simulink model "Model_02"  (R2014a)
settings: Solver=ode3  SolverMode=SingleTasking  StartTime=0.0  StopTime=totalSimulationTime  FixedStep=t_Sim  RelTol=1e-3
model workspace: external: MATLAB File Init_Model_02_Simulink.m (data not in the file)
values from neighbouring files (symbols this model uses):
  Cov_nu = [0.005 0 0 0 ... (first row only)    [InitOOSM.m]    (also in InitSIL.m; Init_Model_02_Simulink.m = 5e-3*eye(4,4); Init_Model_02_Simulink_SIL1.m)
  Cov_r = [0.003 0 0 ... (first row only)    [InitOOSM.m]    (also in InitSIL.m; Init_Model_02_Simulink.m = 3e-3*eye(3,3); Init_Model_02_Simulink_SIL1.m)
  e_force_x = 0    [InitOOSM.m]    (also in InitSIL.m; Init_Model_02_Simulink.m; Init_Model_02_Simulink_SIL1.m)
  e_force_y = 0    [InitOOSM.m]    (also in InitSIL.m; Init_Model_02_Simulink.m; Init_Model_02_Simulink_SIL1.m)
  e_force_z = 0    [InitOOSM.m]    (also in InitSIL.m; Init_Model_02_Simulink.m; Init_Model_02_Simulink_SIL1.m)
  ita = [0.5;0.5;0.5;0.5]    [InitOOSM.m]    (also in InitSIL.m; Init_Model_02_Simulink.m = [0.12;0.05;-0.15;0.98]; Init_Model_02_Simulink_SIL1.m)
  n = 0.00    (= 0)    [InitOOSM.m]    (also in InitSIL.m; Init_Model_02_Simulink_SIL1.m)
  p_x = 0.75    [InitOOSM.m]    (also in InitSIL.m; Init_Model_02_Simulink.m; Init_Model_02_Simulink_SIL1.m)
  p_y = 0.125    [InitOOSM.m]    (also in InitSIL.m; Init_Model_02_Simulink.m; Init_Model_02_Simulink_SIL1.m)
  p_z = -0.8    [InitOOSM.m]    (also in InitSIL.m; Init_Model_02_Simulink.m; Init_Model_02_Simulink_SIL1.m)
  parameter_gravitation = 3.986005E+14    (= 398600500000000)    [InitOOSM.m]    (also in InitSIL.m; Init_Model_02_Simulink_SIL1.m)
  rho = [0.04;0;0.3]    [InitOOSM.m]    (also in InitSIL.m; Init_Model_02_Simulink.m = [0.2;0.1;0.05]; Init_Model_02_Simulink_SIL1.m)
  rho_c = [-0.00017;   -0.9780;   -0.1854]    [InitOOSM.m]    (also in InitSIL.m = [0.00036;   -0.9865;   -0.1854]; Init_Model_02_Simulink.m = [0;0;0.9]; Init_Model_02_Simulink_SIL1.m = [0.00036;   -0.9865;   -0.1854])
  sig_f = 2E-6    (= 2e-06)    [InitOOSM.m]    (also in InitSIL.m; Init_Model_02_Simulink.m; Init_Model_02_Simulink_SIL1.m)
  sig_tau = 2.5E-5    (= 2.5e-05)    [InitOOSM.m]    (also in InitSIL.m; Init_Model_02_Simulink.m; Init_Model_02_Simulink_SIL1.m)
  t_delta = 0.2    [InitOOSM.m]    (also in InitSIL.m; Init_Model_02_Simulink_SIL1.m)
  t_Kalman = 0.01    [InitOOSM.m]    (also in InitSIL.m; Init_Model_02_Simulink_SIL1.m)
  t_Sim = 0.001    [InitOOSM.m]    (also in InitSIL.m; Init_Model_02_Simulink_SIL1.m)
  tau_1 = 0    [InitOOSM.m]    (also in InitSIL.m; Init_Model_02_Simulink.m; Init_Model_02_Simulink_SIL1.m)
  tau_2 = 0    [InitOOSM.m]    (also in InitSIL.m; Init_Model_02_Simulink.m; Init_Model_02_Simulink_SIL1.m)
  tau_3 = 0    [InitOOSM.m]    (also in InitSIL.m; Init_Model_02_Simulink.m; Init_Model_02_Simulink_SIL1.m)
  X_a_0 = [0; 0; 0; 1; 0; 0; 0; 0; 0; 0; 0; 0; 0;0;0;0;0;0;0;1]    [InitOOSM.m]    (also in InitSIL.m = [0; 0; 0; 1; 0; 0; 0; 0; 0; 0; 0; 0; 0]; Init_Model_02_Simulink.m = [q_1_0;q_2_0;q_3_0;q_0_0;om_x_0;om_y_0;om_z_0;r_x_0;r_y_0;r_; Init_Model_02_Simulink_SIL1.m = [0;0;0.707;0.707;0.2;-0.02;0.0001;0.02;-1.80;0.50;-0.05;0.00)
undefined symbols (not defined in the file or in its folder): DiscIntNeverNeededParam, gray
libraries: simulink x7, aerolibtransform2 x2, visionsinks x1
(part 1 of 3)
settings Model: PauseTimes=3  NumberOfSteps=100  Creator=Iseberg-2  LastModifiedBy=Iseberg
settings SolverCC: AutoInsertRateTranBlk=on
settings DebuggingCC: UnderspecifiedInitializationDetection=Classic  CheckExecutionContextPreStartOutputMsg=on  CheckExecutionContextRuntimeOutputMsg=on

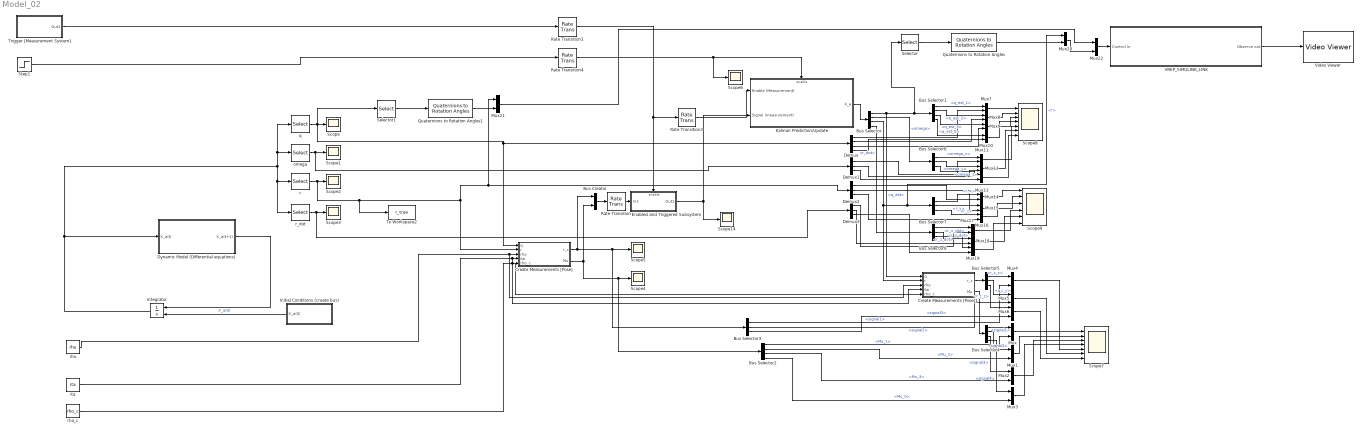
== system Model_02 ==
  Bus Creator : BusCreator  Inputs=2
  Bus Selector : BusSelector  OutputSignals=q_est,omega,r,r_dot
  Bus Selector1 : BusSelector  OutputSignals=q_est_1,q_est_2,q_est_3,q_est_0
  Bus Selector2 : BusSelector  OutputSignals=Mu_1,Mu_2,Mu_3,Mu_0
  Bus Selector3 : BusSelector
  Bus Selector4 : BusSelector  OutputSignals=signal1,signal2,signal3,signal4
  Bus Selector5 : BusSelector  OutputSignals=r_c_x,r_c_y,r_c_z
  Bus Selector6 : BusSelector  OutputSignals=omega_x,omega_y,omega_z
  Bus Selector7 : BusSelector  OutputSignals=r_x,r_y,r_z
  Bus Selector8 : BusSelector  OutputSignals=r_x_dot,r_y_dot,r_z_dot
  Create Measurements [Pose] : Subsystem
  Create Measurements [Pose]1 : Subsystem
  Demux : Demux
  Demux1 : Demux  Outputs=3
  Demux2 : Demux  Outputs=3
  Demux3 : Demux  Outputs=3
  Dynamic Model (Differential equations) : Subsystem
  Enabled and Triggered Subsystem : Subsystem  TreatAsAtomicUnit=on
  Initial Conditions (create bus) : Subsystem
  Integrator : Integrator  InitialConditionSource=external
  Kalman Prediction/Update : Subsystem  TreatAsAtomicUnit=on
  Mux{,1..22} (23 alike) : Mux  Inputs=2
  Quaternions to Rotation Angles : aerolibtransform2/Quaternions to Rotation Angles  rotationOrder=ZYX
  Quaternions to Rotation Angles1 : aerolibtransform2/Quaternions to Rotation Angles  rotationOrder=ZYX
  Rate Transition : RateTransition  OutPortSampleTime=t_delta
  Rate Transition1 : RateTransition  OutPortSampleTime=t_Kalman
  Rate Transition3 : RateTransition  OutPortSampleTime=t_delta
  Rate Transition4 : RateTransition  OutPortSampleTime=t_Kalman
  Scope{,1..6,14} (8 alike) : Scope
      Scope settings: ShowLegends=on  YMin=-1  YMax=1  MaxDataPoints=100000
      Scope1 settings: ShowLegends=on  TimeRange=40
      Scope14 settings: SaveName=ScopeData31
      Scope2 settings: ShowLegends=on  SaveName=ScopeData2
      Scope3 settings: ShowLegends=on  SaveName=ScopeData3
      Scope4 settings: ShowLegends=on  TimeRange=40  SaveName=ScopeData4
      Scope5 settings: ShowLegends=on  SaveName=ScopeData5
      Scope6 settings: YMin=0.95  YMax=1.05  SaveName=ScopeData7
  Scope7 : Scope  NumInputPorts=7
      settings: ShowLegends=on  TimeRange=200  YMin=-1~-5~-5~-5~-5~-5~-5  YMax=1~5~5~5~5~5~5  SaveName=ScopeData9
  Scope8 : Scope  NumInputPorts=7
      settings: ShowLegends=on  TimeRange=200  YMin=-1~-1~-1~-1~0.4~-0.4~-1  YMax=0.75~1~1~0.75~0.95~0.4~1  SaveName=ScopeData24
  Scope9 : Scope  NumInputPorts=6
      settings: ShowLegends=on  TimeRange=200  YMin=-1~-5~-5~-5~-5~-5  YMax=1~5~5~5~5~5  SaveName=ScopeData11
  Selector : Selector  InputPortWidth=4  Indices=[4 1 2 3]
  Selector1 : Selector  InputPortWidth=4  Indices=[4 1 2 3]
  Step1 : Step  Time=0  SampleTime=t_Sim
  To Workspace2 : ToWorkspace  VariableName=r_true  SaveFormat=Timeseries  SampleTime=-1
  Trigger [Measurement System] : Subsystem
  VREP_SIMULINK_LINK : Subsystem  mask{ObjectsInScene=DefaultCamera, m_ControlObjects={ 'Satellite_Model','Parent';'Satellite_Model_Est','Parent'}, m_InitialControllablePose={[X_a_0_sim.X_a_0_Model_02(9:11);X_a_0_sim.eulerAngles_X_a_0'];zeros(6,1)}, m_ObserveObjects={ 'Vision_sensor','Image' }, sceneFileName=C:\Program Files (x86)\V-REP3\V-REP_PRO_EDU\scenes\Scene_MotionEstimation_1.ttt, OutPortSampleTime=0.05}
      mask prompts: ObjectsInScene "Objects present in scene:"; m_ControlObjects "Control Objects:"; m_InitialControllablePose "Initial Pose:"; m_ObserveObjects "Observing Objects:"; sceneFileName "Scene filename:"; OutPortSampleTime "VREP Sample time [s]"
      mask TypeOptions ObjectsInScene: DefaultCamera | DefaultXViewCamera | DefaultYViewCamera | DefaultZViewCamera | XYZCameraProxy | DefaultNXViewCamera | DefaultNYViewCamera | DefaultNZViewCamera | DefaultLightA | DefaultLightB | DefaultLightC | DefaultLightD | ResizableFloor_5_25 | ResizableFloor_5_25_element | ResizableFloor_5_25_visibleElement | Satellite_Model | Satellite_Model_Est | redundantRobot0 | redundantRob_manipSphere0 | redundantRob_target0 | redundantRob_link8 | redundantRob_joint8 | Rectangle0 | redundantRob_joint9 | Cylinder4 | redundantRob_joint10 | Rectangle5 | redundantRob_joint11 | Cylinder5 | redundantRob_joint12 | Rectangle6 | redundantRob_joint13 | Cylinder6 | redundantRob_joint14 | Rectangle7 | redundantRob_link9 | redundantRob_tip0 | redundantRob_link10 | redundantRob_link11 | redundantRob_link12 | redundantRob_link13 | redundantRob_link14 | redundantRob_link15 | Vision_sensor
      mask TypeOptions m_ControlObjects: VREP_SIMULINK_SYS_OBJ/m_ControlObjects
      mask TypeOptions m_InitialControllablePose: VREP_SIMULINK_SYS_OBJ/m_InitialControllablePose
      mask TypeOptions m_ObserveObjects: VREP_SIMULINK_SYS_OBJ/m_ObserveObjects
      mask TypeOptions sceneFileName: VREP_SIMULINK_SYS_OBJ/sceneFileName
      mask TypeOptions OutPortSampleTime: Rate Transition/OutPortSampleTime | Rate Transition1/OutPortSampleTime
      mask DialogControl Control1 Prompt: V-REP Simulink LINK block settings
      mask DialogControl Container8 Prompt: V-REP settings
      mask Display:
      | image('C:\Users\Iseberg\Pictures\Vrep_image.png')
      | port_label('input',1,'Control in');
      | port_label('output',1,'Observe out');
  Video Viewer : visionsinks/Video Viewer  inputType=Obsolete7b  imagePorts=One multidimensional signal  useColorMap=off  colormapValue=gray(256)  specRange=off  minInputVal=0  maxInputVal=255  FigPos=[9 718 1350 611]  AxisZoom=on  trueSizedOnce=off  OpenAtMdlStart=on  DefaultConfigurationName=vipscopes.VideoViewerScopeCfg
  ita : Constant  Value=ita
  omega : Selector  NumberOfDimensions=2  InputPortWidth=3  IndexOptions=Index vector (dialog),Index vector (dialog)  Indices=[5 6 7],1  OutputSizes=1,1
  q : Selector  NumberOfDimensions=2  InputPortWidth=3  IndexOptions=Index vector (dialog),Index vector (dialog)  Indices=[1 2 3 4],1  OutputSizes=1,1
  r : Selector  NumberOfDimensions=2  InputPortWidth=3  IndexOptions=Index vector (dialog),Index vector (dialog)  Indices=[8 9 10],1  OutputSizes=1,1
  r_dot : Selector  NumberOfDimensions=2  InputPortWidth=3  IndexOptions=Index vector (dialog),Index vector (dialog)  Indices=[11 12 13],1  OutputSizes=1,1
  "rho " : Constant  Value=rho
  rho_c : Constant  Value=rho_c
  wires:
  Initial Conditions (create bus)/1("X_a(0) ") -> Integrator/2  "X_a(0)"
  Dynamic Model (Differential equations)/1(X_a(t+1)) -> Integrator/1
  omega/1 -> Demux1/1, Scope1/1
  r_dot/1 -> Demux3/1, Scope3/1
  Integrator/1 -> r_dot/1, r/1, q/1, omega/1, Dynamic Model (Differential equations)/1(X_a(t))
  "rho "/1 -> Create Measurements [Pose]1/3(rho), Create Measurements [Pose]/3(rho)
  ita/1 -> Create Measurements [Pose]1/4(ita), Create Measurements [Pose]/4(ita)
  rho_c/1 -> Create Measurements [Pose]1/5("rho_c "), Create Measurements [Pose]/5("rho_c ")
  Create Measurements [Pose]/1(r_c) -> Bus Selector3/1, Scope5/1, Bus Creator/1
  Create Measurements [Pose]/2(Mu) -> Bus Creator/2, Bus Selector2/1, Scope4/1
  Bus Creator/1 -> Rate Transition/1
  Trigger [Measurement System]/1(Out1) -> Rate Transition1/1
  Kalman Prediction/Update/1(X_a) -> Bus Selector/1
  Bus Selector/1 -> Selector/1, Bus Selector1/1, Create Measurements [Pose]1/1(q)  "<q_est>"
  Bus Selector/3 -> Create Measurements [Pose]1/2(r), Mux20/1, Bus Selector7/1  "<r>"
  Step1/1 -> Rate Transition4/1
  Create Measurements [Pose]1/2(Mu) -> Bus Selector4/1
  Rate Transition1/1 -> Rate Transition3/1, Enabled and Triggered Subsystem/Enable
  Rate Transition3/1 -> Kalman Prediction/Update/1(Enable (Measurement))
  Rate Transition4/1 -> Scope6/1, Kalman Prediction/Update/Enable
  Rate Transition/1 -> Enabled and Triggered Subsystem/1(In1)
  Enabled and Triggered Subsystem/1(Out1) -> Kalman Prediction/Update/2(Signal (measurement)), Scope14/1
  Bus Selector2/1 -> Mux/2  "<Mu_1>"
  Bus Selector4/1 -> Mux/1  "<signal1>"
  Bus Selector4/2 -> Mux1/1  "<signal2>"
  Bus Selector2/2 -> Mux1/2  "<Mu_2>"
  Bus Selector4/3 -> Mux2/1  "<signal3>"
  Bus Selector2/3 -> Mux2/2  "<Mu_3>"
  Bus Selector4/4 -> Mux3/1  "<signal4>"
  Bus Selector2/4 -> Mux3/2  "<Mu_0>"
  Mux/1 -> Scope7/1
  Mux1/1 -> Scope7/2
  Mux2/1 -> Scope7/3
  Mux3/1 -> Scope7/4
  Create Measurements [Pose]1/1(r_c) -> Bus Selector5/1
  Bus Selector5/1 -> Mux4/1  "<r_c_x>"
  Bus Selector3/1 -> Mux4/2  "<signal1>"
  Bus Selector5/2 -> Mux5/1  "<r_c_y>"
  Bus Selector3/2 -> Mux5/2  "<signal2>"
  Bus Selector5/3 -> Mux6/1  "<r_c_z>"
  Bus Selector3/3 -> Mux6/2  "<signal3>"
  Mux4/1 -> Scope7/5
  Mux5/1 -> Scope7/6
  Mux6/1 -> Scope7/7
  Bus Selector1/1 -> Mux7/1  "<q_est_1>"
  Mux7/1 -> Scope8/1
  Demux/1 -> Mux7/2
  q/1 -> Selector1/1, Create Measurements [Pose]/1(q), Demux/1, Scope/1
  Bus Selector1/2 -> Mux8/1  "<q_est_2>"
  Demux/2 -> Mux8/2
  Bus Selector1/3 -> Mux9/1  "<q_est_3>"
  Demux/3 -> Mux9/2
  Bus Selector1/4 -> Mux10/1  "<q_est_0>"
  Demux/4 -> Mux10/2
  Mux8/1 -> Scope8/2
  Mux9/1 -> Scope8/3
  Mux10/1 -> Scope8/4
  Bus Selector/2 -> Bus Selector6/1  "<omega>"
  Bus Selector6/1 -> Mux11/1  "<omega_x>"
  Demux1/1 -> Mux11/2
  Bus Selector6/2 -> Mux12/1  "<omega_y>"
  Demux1/2 -> Mux12/2
  Bus Selector6/3 -> Mux13/1  "<omega_z>"
  Demux1/3 -> Mux13/2
  Mux11/1 -> Scope8/5
  Mux12/1 -> Scope8/6
  Mux13/1 -> Scope8/7
  Bus Selector7/1 -> Mux14/1  "<r_x>"
  Demux2/1 -> Mux14/2
  Bus Selector7/2 -> Mux15/1  "<r_y>"
  Demux2/2 -> Mux15/2
  Bus Selector7/3 -> Mux16/1  "<r_z>"
  Demux2/3 -> Mux16/2
  Mux14/1 -> Scope9/1
  Mux15/1 -> Scope9/2
  Mux16/1 -> Scope9/3
  Bus Selector/4 -> Bus Selector8/1  "<r_dot>"
  Bus Selector8/1 -> Mux17/1  "<r_x_dot>"
  Demux3/1 -> Mux17/2
  Bus Selector8/2 -> Mux18/1  "<r_y_dot>"
  Demux3/2 -> Mux18/2
  Bus Selector8/3 -> Mux19/1  "<r_z_dot>"
  Demux3/3 -> Mux19/2
  Mux17/1 -> Scope9/4
  Mux18/1 -> Scope9/5
  Mux19/1 -> Scope9/6
  Selector/1 -> Quaternions to Rotation Angles/1
  Selector1/1 -> Quaternions to Rotation Angles1/1
  Quaternions to Rotation Angles1/1 -> Mux21/2
  VREP_SIMULINK_LINK/1(Observe out) -> Video Viewer/1
  r/1 -> To Workspace2/1, Create Measurements [Pose]/2(r), Mux21/1, Demux2/1, Scope2/1
  Quaternions to Rotation Angles/1 -> Mux20/2
  Mux21/1 -> Mux22/1
  Mux20/1 -> Mux22/2
  Mux22/1 -> VREP_SIMULINK_LINK/1(Control In)

== system Model_02/Create Measurements [Pose] ==
  q : Inport
  r : Inport  Port=2
  rho : Inport  Port=3
  ita : Inport  Port=4
  "rho_c " : Inport  Port=5
  "Create Measurements [Orientation] " : Subsystem
  Create Measurements [Position] : Subsystem
  r_c : Outport
  Mu : Outport  Port=2
  wires:
  "rho_c "/1 -> Create Measurements [Position]/4("rho_c ")
  rho/1 -> Create Measurements [Position]/3(rho)
  Create Measurements [Position]/1(r_c) -> r_c/1
  ita/1 -> "Create Measurements [Orientation] "/2("ita ")
  "Create Measurements [Orientation] "/1(Mu) -> Mu/1
  r/1 -> Create Measurements [Position]/1(r)
  q/1 -> Create Measurements [Position]/2(q), "Create Measurements [Orientation] "/1(q)

== system Model_02/Create Measurements [Pose]1 ==
  q : Inport
  r : Inport  Port=2
  rho : Inport  Port=3
  ita : Inport  Port=4
  "rho_c " : Inport  Port=5
  "Create Measurements [Orientation] " : Subsystem
  Create Measurements [Position] : Subsystem
  Rate Transition : RateTransition
  Rate Transition1 : RateTransition
  Rate Transition2 : RateTransition
  r_c : Outport
  Mu : Outport  Port=2
  wires:
  q/1 -> "Create Measurements [Orientation] "/1(q), Create Measurements [Position]/2(q)
  r/1 -> Create Measurements [Position]/1(r)
  "Create Measurements [Orientation] "/1(Mu) -> Mu/1
  ita/1 -> Rate Transition1/1
  Create Measurements [Position]/1(r_c) -> r_c/1
  rho/1 -> Rate Transition2/1
  "rho_c "/1 -> Rate Transition/1
  Rate Transition/1 -> Create Measurements [Position]/4("rho_c ")
  Rate Transition1/1 -> "Create Measurements [Orientation] "/2("ita ")
  Rate Transition2/1 -> Create Measurements [Position]/3(rho)

== system Model_02/Dynamic Model (Differential equations) ==
  X_a(t) : Inport
  Bus Creator : BusCreator
  Constant : Constant  Value=[0]
  "Orbital Dynamics " : Subsystem
  Quaternion Kinematics : Subsystem
  Rotational Dynamics : Subsystem
  Vector Concatenate : Concatenate
  n : Constant  Value=n
  omega : Selector  NumberOfDimensions=2  InputPortWidth=3  IndexOptions=Index vector (dialog),Index vector (dialog)  Indices=[5 6 7],1  OutputSizes=1,1
  p : Constant  Value=[p_x;p_y;p_z]
  parameter_gravitation : Constant  Value=parameter_gravitation
  q : Selector  NumberOfDimensions=2  InputPortWidth=3  IndexOptions=Index vector (dialog),Index vector (dialog)  Indices=[1 2 3 4],1  OutputSizes=1,1
  r : Selector  NumberOfDimensions=2  InputPortWidth=3  IndexOptions=Index vector (dialog),Index vector (dialog)  Indices=[8 9 10],1  OutputSizes=1,1
  r_dot : Selector  NumberOfDimensions=2  InputPortWidth=3  IndexOptions=Index vector (dialog),Index vector (dialog)  Indices=[11 12 13],1  OutputSizes=1,1
  X_a(t+1) : Outport
  wires:
  Constant/1 -> Vector Concatenate/2
  p/1 -> Rotational Dynamics/2(p)
  Vector Concatenate/1 -> Quaternion Kinematics/2(omega_rel)
  parameter_gravitation/1 -> "Orbital Dynamics "/2(Mu)
  n/1 -> "Orbital Dynamics "/3(n)
  "Orbital Dynamics "/1("r_ddot ") -> Bus Creator/4  "r_ddot"
  Quaternion Kinematics/1(q_dot) -> Bus Creator/1  "q_dot"
  Rotational Dynamics/1(omega_dot) -> Bus Creator/2  "omega_dot"
  X_a(t)/1 -> q/1, omega/1, r_dot/1, r/1
  q/1 -> Quaternion Kinematics/1(q)
  omega/1 -> Rotational Dynamics/1(omega), Vector Concatenate/1
  r/1 -> "Orbital Dynamics "/1(r)
  r_dot/1 -> "Orbital Dynamics "/4("r_dot "), Bus Creator/3
  Bus Creator/1 -> X_a(t+1)/1

== system Model_02/Enabled and Triggered Subsystem ==
  In1 : Inport
  Enable : EnablePort  ShowOutputPort=on
  Scope : Scope
      settings: SaveName=ScopeData10
  Out1 : Outport
  wires:
  In1/1 -> Out1/1
  Enable/1 -> Scope/1

== system Model_02/Initial Conditions (create bus) ==
  Bus Creator : BusCreator
  Bus Creator1 : BusCreator  Inputs=3
  Bus Creator2 : BusCreator  Inputs=3
  Bus Creator3 : BusCreator  Inputs=3
  Bus Creator4 : BusCreator
  Demux : Demux  Outputs=13
  Initial conditions (Dynamic Model) : FromFile  FileName=X_a_0_Model_02.mat  SampleTime=0
  "X_a(0) " : Outport
  wires:
  Initial conditions (Dynamic Model)/1 -> Demux/1
  Demux/1 -> Bus Creator/1  "q_1"
  Demux/2 -> Bus Creator/2  "q_2"
  Demux/3 -> Bus Creator/3  "q_3"
  Demux/4 -> Bus Creator/4  "q_0"
  Demux/5 -> Bus Creator1/1  "omega_x"
  Demux/6 -> Bus Creator1/2  "omega_y"
  Demux/7 -> Bus Creator1/3  "omega_z"
  Demux/8 -> Bus Creator2/1  "r_x"
  Demux/9 -> Bus Creator2/2  "r_y"
  Demux/10 -> Bus Creator2/3  "r_z"
  Demux/11 -> Bus Creator3/1  "r_x_dot"
  Demux/12 -> Bus Creator3/2  "r_y_dot"
  Demux/13 -> Bus Creator3/3  "r_z_dot"
  Bus Creator/1 -> Bus Creator4/1  "q"
  Bus Creator1/1 -> Bus Creator4/2  "omega"
  Bus Creator2/1 -> Bus Creator4/3  "r"
  Bus Creator3/1 -> Bus Creator4/4  "r_dot"
  Bus Creator4/1 -> "X_a(0) "/1  "X_a(0)"

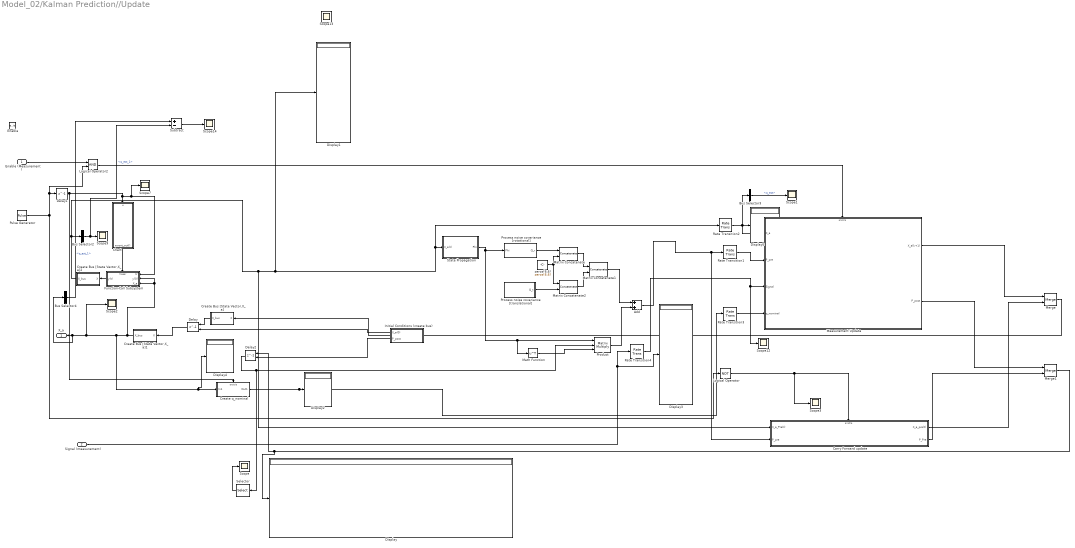
== system Model_02/Kalman Prediction//Update ==
  Enable (Measurement) : Inport
  Signal (measurement) : Inport  Port=2
  Enable : EnablePort  ShowOutputPort=on
  Add : Sum
  Bus Selector2 : BusSelector  OutputSignals=q_est.q_est_1
  Bus Selector3 : BusSelector  OutputSignals=q_est
  Bus Selector4 : BusSelector  OutputSignals=q_est.q_est_1
  Carry Forward update : Subsystem  TreatAsAtomicUnit=on
  Chart : Stateflow chart  TreatAsAtomicUnit=on
  Create Bus [State Vector,X_a] : Subsystem
  Create Bus [State Vector,X_a]1 : Subsystem
  Create Bus [State Vector,X_a]2 : Subsystem
  Create q_nominal : Subsystem  TreatAsAtomicUnit=on
  Delay : Delay  DelayLength=1  InitialConditionSource=Input port  InitialCondition=0  SampleTime=t_Kalman
      settings: InputPortMap=u0,p4
  Delay1 : Delay  DelayLength=1  InitialCondition=0
  Delay2 : Delay  DelayLength=1  InitialConditionSource=Input port  InitialCondition=0  SampleTime=t_Kalman
      settings: InputPortMap=u0,p4
  Display{,1..5} (6 alike) : Display
  Function-Call Subsystem : Subsystem  TreatAsAtomicUnit=on
  Initial Conditions (create bus) : Subsystem
  Logical Operator : Logic  Operator=NOT  AllPortsSameDT=off  OutDataTypeStr=boolean
  Logical Operator2 : Logic  AllPortsSameDT=off  OutDataTypeStr=boolean
  Math Function : Math  Operator=transpose  SaturateOnIntegerOverflow=on
  Matrix Concatenate : Concatenate  Mode=Multidimensional array  ConcatenateDimension=2
  Matrix Concatenate1 : Concatenate  Mode=Multidimensional array
  Matrix Concatenate2 : Concatenate  Mode=Multidimensional array  ConcatenateDimension=2
  Measurement Update : Subsystem  TreatAsAtomicUnit=on
  Merge : Merge  InitialOutput=X_a_0
  Merge1 : Merge  InitialOutput=eye(12,12)
  Process noise covariance [rotational] : Subsystem
  Process noise covariance [translational] : Subsystem
  Product : Product  Inputs=3  Multiplication=Matrix(*)
  Pulse Generator : DiscretePulseGenerator  Period=10  SampleTime=t_Kalman
  Rate Transition{1..4} (4 alike) : RateTransition  OutPortSampleTime=t_delta
  Scope{,1..3,7,9,12..14} (9 alike) : Scope
      Scope settings: SaveName=ScopeData38
      Scope1 settings: TimeRange=2.384805435453984  YMin=0.002979591836734694  YMax=0.003650793650793651  SaveName=ScopeData12
      Scope12 settings: ShowLegends=on  YMin=-0.75  YMax=2.75  SaveName=ScopeData34
      Scope13 settings: ShowLegends=on  TimeRange=40  YMin=-1  YMax=1.1  SaveName=ScopeData36
      Scope14 settings: ShowLegends=on  TimeRange=10  YMin=-1  YMax=1  SaveName=ScopeData39
      Scope2 settings: ShowLegends=on  SaveName=ScopeData19
      Scope3 settings: ShowLegends=on  SaveName=ScopeData16
      Scope7 settings: ShowLegends=on  TimeRange=40  SaveName=ScopeData32
      Scope9 settings: ShowLegends=on  TimeRange=40  YMin=-0.2597  YMax=-0.2575  SaveName=ScopeData33
  Selector : Selector  NumberOfDimensions=2  InputPortWidth=3  IndexOptions=Index vector (dialog),Index vector (dialog)  Indices=[4],[4]  OutputSizes=1,1
  State Propagation : Subsystem
  Subtract : Sum  Inputs=+-
  zeros(6,6) : Constant  Value=zeros(6,6)
  X_a : Outport
  wires:
  State Propagation/1(Phi) -> Math Function/1, Product/1, Process noise covariance [rotational]/1(Phi)
  Process noise covariance [rotational]/1(Q_r) -> Matrix Concatenate/1
  zeros(6,6)/1 -> Matrix Concatenate2/1, Matrix Concatenate/2
  Process noise covariance [translational]/1(Q_t) -> Matrix Concatenate2/2
  Matrix Concatenate/1 -> Matrix Concatenate1/1
  Matrix Concatenate2/1 -> Matrix Concatenate1/2
  Math Function/1 -> Product/3
  Matrix Concatenate1/1 -> Add/1
  Product/1 -> Add/2
  Initial Conditions (create bus)/2("P_post ") -> Delay2/2
  Enable (Measurement)/1 -> Logical Operator2/1
  Add/1 -> Carry Forward update/2(P_pre), Rate Transition1/1
  Logical Operator2/1 -> Measurement Update/Enable
  Carry Forward update/2(P_Pre) -> Merge1/2
  Merge1/1 -> Display/1, Delay2/1
  Logical Operator/1 -> Carry Forward update/Enable, Scope3/1
  Carry Forward update/1("X_a_pre(t) ") -> Merge/2
  Signal (measurement)/1 -> Display3/1, Rate Transition4/1
  Rate Transition4/1 -> Scope12/1, Measurement Update/3(Signal)
  Rate Transition2/1 -> Bus Selector3/1, Display5/1, Measurement Update/1(X_a)
  Rate Transition1/1 -> Measurement Update/2(P_pre)
  Measurement Update/1(X_a(k+1)) -> Merge/1
  Measurement Update/2(P_post) -> Merge1/1
  Pulse Generator/1 -> Logical Operator2/2, Delay1/1, Logical Operator/1
  Create Bus [State Vector,X_a]/1(X_bus) -> Delay/1
  Merge/1 -> Create Bus [State Vector,X_a]/1(X)
  Delay1/1 -> Scope7/1, Function-Call Subsystem/1(tr), Chart/1(u), Create q_nominal/Enable
  Selector/1 -> Scope/1
  Delay2/1 -> Selector/1, Product/2
  Chart/1(event_out()) -> Function-Call Subsystem/Trigger
  Function-Call Subsystem/1(y(t)) -> Create Bus [State Vector,X_a]2/1(X)
  Bus Selector2/1 -> Subtract/2, Scope9/1  "<q_est_1>"
  Bus Selector4/1 -> Subtract/1  "<q_est_1>"
  Subtract/1 -> Scope14/1
  Bus Selector3/1 -> Scope1/1  "<q_est>"
  Create Bus [State Vector,X_a]2/1(X_bus) -> Carry Forward update/1(X_a_Pre(t)), Display1/1, Rate Transition2/1, State Propagation/1("X_a(t)\t"), Bus Selector2/1
  Delay/1 -> Create Bus [State Vector,X_a]1/1(X)
  Rate Transition3/1 -> Measurement Update/4("q_nominal ")
  Initial Conditions (create bus)/1("X_a(0) ") -> Delay/2
  Create q_nominal/1(Out1) -> Display2/1, Rate Transition3/1
  Create Bus [State Vector,X_a]1/1(X_bus) -> Function-Call Subsystem/3(X_a), Function-Call Subsystem/2(y(0)), Display4/1, Create q_nominal/1(In1), Scope2/1, Bus Selector4/1, X_a/1

== system Model_02/Trigger [Measurement System] ==
  Add : Sum  Inputs=+++
  Step : Step  Time=3  SampleTime=t_Sim
  Step1 : Step  Time=25  After=-1  SampleTime=t_Sim
  Step2 : Step  Time=35  SampleTime=t_Sim
  Out1 : Outport
  wires:
  Add/1 -> Out1/1
  Step/1 -> Add/2
  Step1/1 -> Add/1
  Step2/1 -> Add/3

== system Model_02/VREP_SIMULINK_LINK ==
  Control In : Inport
  Rate Transition : RateTransition  OutPortSampleTime=OutPortSampleTime
  Rate Transition1 : RateTransition  OutPortSampleTime=OutPortSampleTime
  VREP_SIMULINK_SYS_OBJ : MATLABSystem  System=SysObjVREP_1  SimulateUsing=Interpreted execution  ObjectsInScene=''  sceneFileName=C:\Program Files (x86)\V-REP3\V-REP_PRO_EDU\scenes\Scene_MotionEstimation_1.ttt  m_ControlObjects=m_ControlObjects  m_ObserveObjects=m_ObserveObjects  m_InitialControllablePose=m_InitialControllablePose
      mask Type: SysObjVREP_1
      mask Display:
      | disp('V-REP');
      | port_label('input',1,'ControlPose(2)');
      | port_label('output',1,'ObservePose(1)');
  Observe out : Outport
  wires:
  Control In/1 -> Rate Transition/1
  VREP_SIMULINK_SYS_OBJ/1 -> Rate Transition1/1
  Rate Transition/1 -> VREP_SIMULINK_SYS_OBJ/1
  Rate Transition1/1 -> Observe out/1

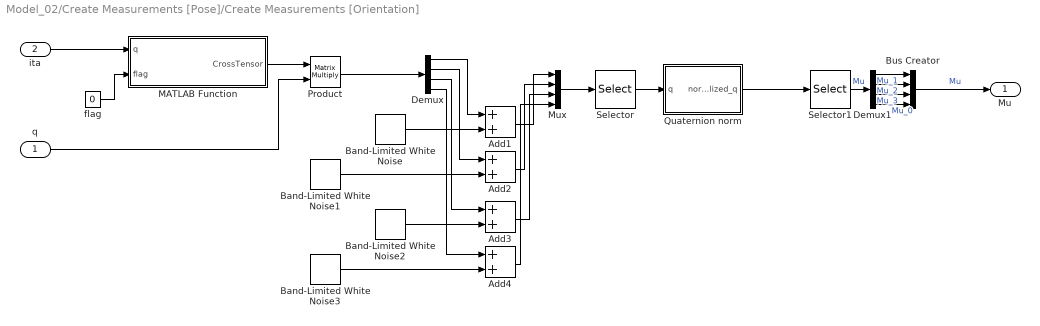
== system Model_02/Create Measurements [Pose]/Create Measurements [Orientation]  ==
  q : Inport
  "ita " : Inport  Port=2
  Add{1..4} (4 alike) : Sum
  Band-Limited White Noise : simulink/Sources/Band-Limited White Noise  Cov=[0.000001]  Ts=t_Kalman  seed=[13441]
  Band-Limited White Noise1 : simulink/Sources/Band-Limited White Noise  Cov=[0.000001]  Ts=t_Kalman  seed=[43321]
  Band-Limited White Noise2 : simulink/Sources/Band-Limited White Noise  Cov=[0.000001]  Ts=t_Kalman  seed=[24321]
  Band-Limited White Noise3 : simulink/Sources/Band-Limited White Noise  Cov=[0.000001]  Ts=t_Kalman  seed=[12345]
  Bus Creator : BusCreator
  Demux : Demux
  Demux1 : Demux
  MATLAB Function : MATLAB Function  TreatAsAtomicUnit=on
  Mux : Mux
  Product : Product  Multiplication=Matrix(*)
  Quaternion norm : Subsystem
  Selector : Selector  NumberOfDimensions=2  InputPortWidth=3  IndexOptions=Index vector (dialog),Index vector (dialog)  Indices=[4 1 2 3],1  OutputSizes=1,1
  Selector1 : Selector  NumberOfDimensions=2  InputPortWidth=3  IndexOptions=Index vector (dialog),Index vector (dialog)  Indices=[2 3 4 1],1  OutputSizes=1,1
  "flag " : Constant  Value=0
  Mu : Outport
  wires:
  Selector/1 -> Quaternion norm/1(q)
  "flag "/1 -> MATLAB Function/2(flag)
  MATLAB Function/1(CrossTensor) -> Product/1
  "ita "/1 -> MATLAB Function/1(q)
  Quaternion norm/1(normalized_q) -> Selector1/1
  Mux/1 -> Selector/1
  Add3/1 -> Mux/3
  Demux/3 -> Add3/1
  Demux/1 -> Add1/1
  Demux/4 -> Add4/1
  Add1/1 -> Mux/1
  Add2/1 -> Mux/2
  Add4/1 -> Mux/4
  Demux1/4 -> Bus Creator/4  "Mu_0"
  Selector1/1 -> Demux1/1  "Mu"
  Demux1/1 -> Bus Creator/1  "Mu_1"
  Demux1/2 -> Bus Creator/2  "Mu_2"
  Demux1/3 -> Bus Creator/3  "Mu_3"
  Bus Creator/1 -> Mu/1  "Mu"
  q/1 -> Product/2
  Product/1 -> Demux/1
  Demux/2 -> Add2/1
  Band-Limited White Noise/1 -> Add1/2
  Band-Limited White Noise1/1 -> Add2/2
  Band-Limited White Noise2/1 -> Add3/2
  Band-Limited White Noise3/1 -> Add4/2

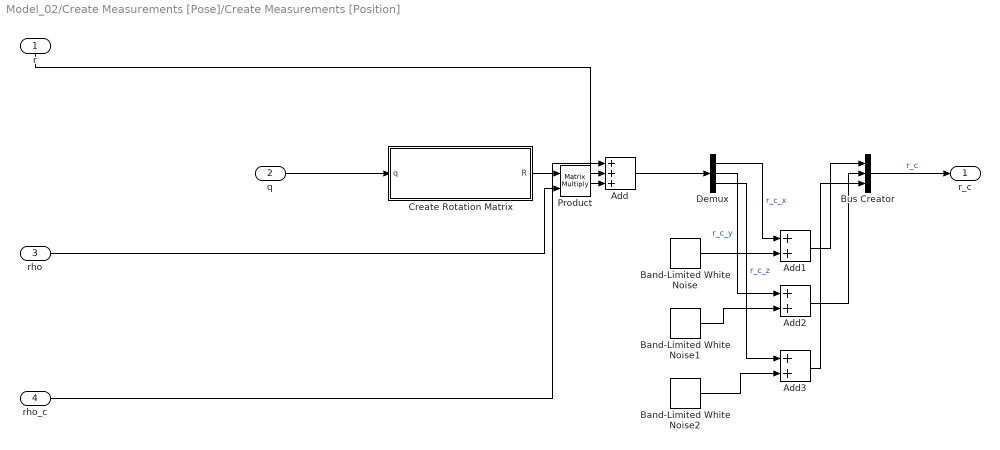
== system Model_02/Create Measurements [Pose]/Create Measurements [Position] ==
  r : Inport
  q : Inport  Port=2
  rho : Inport  Port=3
  "rho_c " : Inport  Port=4
  Add : Sum  Inputs=+++
  Add1 : Sum
  Add2 : Sum
  Add3 : Sum
  Band-Limited White Noise : simulink/Sources/Band-Limited White Noise  Cov=[0.0001]  Ts=t_Kalman  seed=[23341]
  Band-Limited White Noise1 : simulink/Sources/Band-Limited White Noise  Cov=[0.0001]  Ts=t_Kalman  seed=[43321]
  Band-Limited White Noise2 : simulink/Sources/Band-Limited White Noise  Cov=[0.0001]  Ts=t_Kalman  seed=[12342]
  Bus Creator : BusCreator  Inputs=3
  "Create Rotation Matrix " : Subsystem
  Demux : Demux  Outputs=3
  Product : Product  Multiplication=Matrix(*)
  r_c : Outport
  wires:
  Product/1 -> Add/3
  "Create Rotation Matrix "/1(R) -> Product/1
  Demux/1 -> Add1/1  "r_c_x"
  rho/1 -> Product/2
  "rho_c "/1 -> Add/1
  q/1 -> "Create Rotation Matrix "/1(q)
  Demux/3 -> Add3/1  "r_c_z"
  Demux/2 -> Add2/1  "r_c_y"
  Bus Creator/1 -> r_c/1  "r_c"
  r/1 -> Add/2
  Add1/1 -> Bus Creator/1
  Add2/1 -> Bus Creator/2
  Add3/1 -> Bus Creator/3
  Add/1 -> Demux/1
  Band-Limited White Noise/1 -> Add1/2
  Band-Limited White Noise1/1 -> Add2/2
  Band-Limited White Noise2/1 -> Add3/2

== system Model_02/Create Measurements [Pose]1/Create Measurements [Orientation]  ==
  q : Inport
  "ita " : Inport  Port=2
  Bus Creator : BusCreator
  Demux : Demux
  MATLAB Function : MATLAB Function  TreatAsAtomicUnit=on
  Product : Product  Multiplication=Matrix(*)
  "flag " : Constant  Value=0
  Mu : Outport
  wires:
  Product/1 -> Demux/1
  q/1 -> Product/2
  Bus Creator/1 -> Mu/1  "Mu"
  "ita "/1 -> MATLAB Function/1(q)
  MATLAB Function/1(CrossTensor) -> Product/1
  "flag "/1 -> MATLAB Function/2(flag)
  Demux/1 -> Bus Creator/1
  Demux/2 -> Bus Creator/2
  Demux/3 -> Bus Creator/3
  Demux/4 -> Bus Creator/4

== system Model_02/Create Measurements [Pose]1/Create Measurements [Position] ==
  r : Inport
  q : Inport  Port=2
  rho : Inport  Port=3
  "rho_c " : Inport  Port=4
  Add : Sum  Inputs=+++
  Bus Creator : BusCreator  Inputs=3
  "Create Rotation Matrix " : Subsystem
  Demux : Demux  Outputs=3
  Product : Product  Multiplication=Matrix(*)
  r_c : Outport
  wires:
  Add/1 -> Demux/1
  r/1 -> Add/2
  Bus Creator/1 -> r_c/1  "r_c"
  q/1 -> "Create Rotation Matrix "/1(q)
  "rho_c "/1 -> Add/1
  rho/1 -> Product/2
  "Create Rotation Matrix "/1(R) -> Product/1
  Product/1 -> Add/3
  Demux/1 -> Bus Creator/1  "r_c_x"
  Demux/2 -> Bus Creator/2  "r_c_y"
  Demux/3 -> Bus Creator/3  "r_c_z"

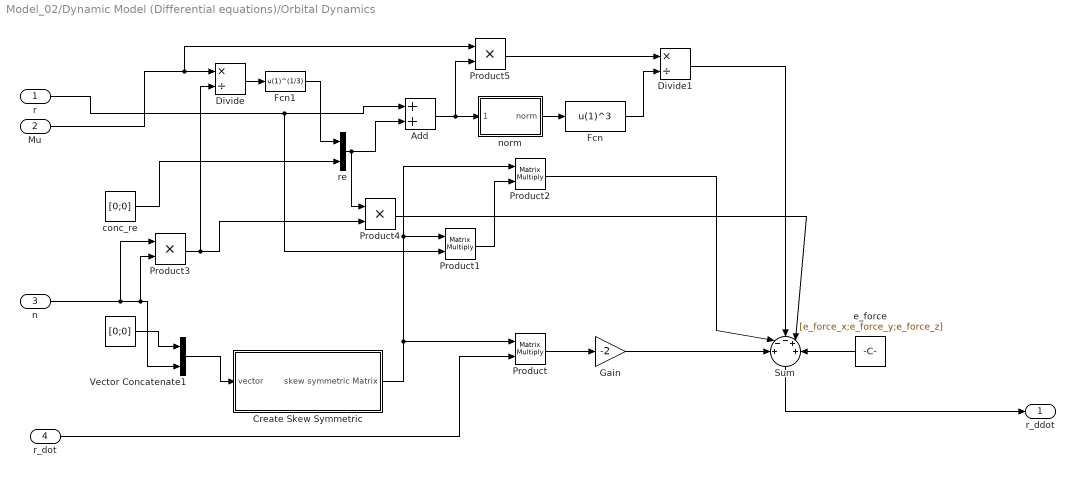
== system Model_02/Dynamic Model (Differential equations)/Orbital Dynamics  ==
  r : Inport
  Mu : Inport  Port=2
  n : Inport  Port=3
  "r_dot " : Inport  Port=4
  " " : Constant  Value=[0;0]
  Add : Sum
  Create Skew Symmetric : Subsystem
  Divide : Product  Inputs=*/
  Divide1 : Product  Inputs=*/
  Fcn : Fcn  Expr=u(1)^3
  Fcn1 : Fcn  Expr=u(1)^(1/3)
  Gain : Gain  Gain=-2
  Product : Product  Multiplication=Matrix(*)
  Product1 : Product  Multiplication=Matrix(*)
  Product2 : Product  Multiplication=Matrix(*)
  Product3 : Product
  Product4 : Product
  Product5 : Product
  Sum : Sum  Inputs=+--++
  Vector Concatenate1 : Concatenate
  "conc_re " : Constant  Value=[0;0]
  "e_force " : Constant  Value=[e_force_x;e_force_y;e_force_z]
  "norm " : Subsystem
  re : Concatenate
  "r_ddot " : Outport
  wires:
  " "/1 -> Vector Concatenate1/1
  Create Skew Symmetric/1(skew symmetric Matrix) -> Product/1, Product1/1, Product2/1
  Product1/1 -> Product2/2
  Mu/1 -> Product5/1, Divide/1
  Product/1 -> Gain/1
  "conc_re "/1 -> re/2
  re/1 -> Product4/1, Add/2
  Product5/1 -> Divide1/1
  "norm "/1("norm ") -> Fcn/1
  n/1 -> Product3/2, Vector Concatenate1/2, Product3/1
  Product3/1 -> Divide/2, Product4/2
  Vector Concatenate1/1 -> Create Skew Symmetric/1(vector)
  Add/1 -> "norm "/1(vector), Product5/2
  Gain/1 -> Sum/1
  Product2/1 -> Sum/2
  r/1 -> Product1/2, Add/1
  Product4/1 -> Sum/4
  "r_dot "/1 -> Product/2
  Divide1/1 -> Sum/3
  Fcn1/1 -> re/1
  Fcn/1 -> Divide1/2
  Divide/1 -> Fcn1/1
  "e_force "/1 -> Sum/5
  Sum/1 -> "r_ddot "/1

== system Model_02/Dynamic Model (Differential equations)/Quaternion Kinematics ==
  q : Inport
  omega_rel : Inport  Port=2
  Constant2 : Constant  Value=0.5
  MATLAB Function : MATLAB Function  TreatAsAtomicUnit=on
  Product : Product  Multiplication=Matrix(*)
  Product1 : Product
  flag : Constant
  q_dot : Outport
  wires:
  MATLAB Function/1(CrossTensor) -> Product/1
  flag/1 -> MATLAB Function/2(flag)
  Constant2/1 -> Product1/2
  q/1 -> MATLAB Function/1(q)
  omega_rel/1 -> Product/2
  Product1/1 -> q_dot/1
  Product/1 -> Product1/1

== system Model_02/Dynamic Model (Differential equations)/Rotational Dynamics ==
  omega : Inport
  p : Inport  Port=2
  Add : Sum
  Create  J : Subsystem
  Create Psi : Subsystem
  Product : Product  Multiplication=Matrix(*)
  tau : Constant  Value=[tau_1;tau_2;tau_3]
  omega_dot : Outport
  wires:
  omega/1 -> Create Psi/1("omega ")
  Create Psi/1(Psi) -> Add/1
  Add/1 -> omega_dot/1
  Product/1 -> Add/2
  p/1 -> Create Psi/2(p), Create  J/1(p)
  Create  J/1("J_k ") -> Product/1
  tau/1 -> Product/2

== system Model_02/Kalman Prediction//Update/Carry Forward update ==
  X_a_Pre(t) : Inport
  P_pre : Inport  Port=2
  Enable : EnablePort
  "X_a_pre(t) " : Outport
  P_Pre : Outport  Port=2
  wires:
  X_a_Pre(t)/1 -> "X_a_pre(t) "/1
  P_pre/1 -> P_Pre/1

== system Model_02/Kalman Prediction//Update/Chart/S.Integ ==
  u : Inport  OutDataTypeStr=double  PortDimensions=1
  tr : Inport  Port=2  OutDataTypeStr=double  PortDimensions=1
  y0 : Inport  Port=3  OutDataTypeStr=double  PortDimensions=1
  f : TriggerPort  TriggerType=function-call
      settings: CopyFcn=Stateflow.SLINSF.SimulinkMan.removeBlockPreDeleteFcn  PreDeleteFcn=Stateflow.SLINSF.SimulinkMan.unsafePredeleteFcn
  Discrete-Time Integrator2 : DiscreteIntegrator  ExternalReset=rising  InitialConditionSource=external  SampleTime=-1  ShowStatePort=on  ICPrevOutput=DiscIntNeverNeededParam  ICPrevScaledInput=DiscIntNeverNeededParam
  y_t : Outport  OutDataTypeStr=double  PortDimensions=1
  wires:
  u/1 -> Discrete-Time Integrator2/1
  tr/1 -> Discrete-Time Integrator2/2
  y0/1 -> Discrete-Time Integrator2/3
  Discrete-Time Integrator2/1 -> y_t/1

== system Model_02/Kalman Prediction//Update/Create Bus [State Vector,X_a] ==
  X : Inport
  Bus Creator2 : BusCreator
  Bus Creator3 : BusCreator  Inputs=3
  Bus Creator4 : BusCreator  Inputs=3
  Bus Creator5 : BusCreator  Inputs=3
  Bus Creator6 : BusCreator
  Demux1 : Demux  Outputs=13
  X_bus : Outport
  wires:
  Bus Creator2/1 -> Bus Creator6/1  "q_est"
  Bus Creator3/1 -> Bus Creator6/2  "omega"
  Bus Creator4/1 -> Bus Creator6/3  "r"
  Bus Creator5/1 -> Bus Creator6/4  "r_dot"
  Bus Creator6/1 -> X_bus/1
  X/1 -> Demux1/1
  Demux1/1 -> Bus Creator2/1  "q_est_1"
  Demux1/2 -> Bus Creator2/2  "q_est_2"
  Demux1/3 -> Bus Creator2/3  "q_est_3"
  Demux1/4 -> Bus Creator2/4  "q_est_0"
  Demux1/5 -> Bus Creator3/1  "omega_x"
  Demux1/6 -> Bus Creator3/2  "omega_y"
  Demux1/7 -> Bus Creator3/3  "omega_z"
  Demux1/8 -> Bus Creator4/1  "r_x"
  Demux1/9 -> Bus Creator4/2  "r_y"
  Demux1/10 -> Bus Creator4/3  "r_z"
  Demux1/11 -> Bus Creator5/1  "r_x_dot"
  Demux1/12 -> Bus Creator5/2  "r_y_dot"
  Demux1/13 -> Bus Creator5/3  "r_z_dot"

== system Model_02/Kalman Prediction//Update/Create Bus [State Vector,X_a]1 ==
  X : Inport
  Bus Creator2 : BusCreator
  Bus Creator3 : BusCreator  Inputs=3
  Bus Creator4 : BusCreator  Inputs=3
  Bus Creator5 : BusCreator  Inputs=3
  Bus Creator6 : BusCreator
  Demux1 : Demux  Outputs=13
  X_bus : Outport
  wires:
  Bus Creator2/1 -> Bus Creator6/1  "q_est"
  Bus Creator3/1 -> Bus Creator6/2  "omega"
  Bus Creator4/1 -> Bus Creator6/3  "r"
  Bus Creator5/1 -> Bus Creator6/4  "r_dot"
  Bus Creator6/1 -> X_bus/1
  X/1 -> Demux1/1
  Demux1/1 -> Bus Creator2/1  "q_est_1"
  Demux1/2 -> Bus Creator2/2  "q_est_2"
  Demux1/3 -> Bus Creator2/3  "q_est_3"
  Demux1/4 -> Bus Creator2/4  "q_est_0"
  Demux1/5 -> Bus Creator3/1  "omega_x"
  Demux1/6 -> Bus Creator3/2  "omega_y"
  Demux1/7 -> Bus Creator3/3  "omega_z"
  Demux1/8 -> Bus Creator4/1  "r_x"
  Demux1/9 -> Bus Creator4/2  "r_y"
  Demux1/10 -> Bus Creator4/3  "r_z"
  Demux1/11 -> Bus Creator5/1  "r_x_dot"
  Demux1/12 -> Bus Creator5/2  "r_y_dot"
  Demux1/13 -> Bus Creator5/3  "r_z_dot"

== system Model_02/Kalman Prediction//Update/Create Bus [State Vector,X_a]2 ==
  X : Inport
  Bus Creator2 : BusCreator
  Bus Creator3 : BusCreator  Inputs=3
  Bus Creator4 : BusCreator  Inputs=3
  Bus Creator5 : BusCreator  Inputs=3
  Bus Creator6 : BusCreator
  Demux1 : Demux  Outputs=13
  X_bus : Outport
  wires:
  Bus Creator2/1 -> Bus Creator6/1  "q_est"
  Bus Creator3/1 -> Bus Creator6/2  "omega"
  Bus Creator4/1 -> Bus Creator6/3  "r"
  Bus Creator5/1 -> Bus Creator6/4  "r_dot"
  Bus Creator6/1 -> X_bus/1
  X/1 -> Demux1/1
  Demux1/1 -> Bus Creator2/1  "q_est_1"
  Demux1/2 -> Bus Creator2/2  "q_est_2"
  Demux1/3 -> Bus Creator2/3  "q_est_3"
  Demux1/4 -> Bus Creator2/4  "q_est_0"
  Demux1/5 -> Bus Creator3/1  "omega_x"
  Demux1/6 -> Bus Creator3/2  "omega_y"
  Demux1/7 -> Bus Creator3/3  "omega_z"
  Demux1/8 -> Bus Creator4/1  "r_x"
  Demux1/9 -> Bus Creator4/2  "r_y"
  Demux1/10 -> Bus Creator4/3  "r_z"
  Demux1/11 -> Bus Creator5/1  "r_x_dot"
  Demux1/12 -> Bus Creator5/2  "r_y_dot"
  Demux1/13 -> Bus Creator5/3  "r_z_dot"

== system Model_02/Kalman Prediction//Update/Create q_nominal ==
  In1 : Inport
  Enable : EnablePort
  Bus Selector1 : BusSelector  OutputSignals=q_est,omega
  Create Bus [State Vector,X_a]3 : Subsystem
  Create nominal q : Subsystem
  Scope6 : Scope
      settings: ShowLegends=on  SaveName=ScopeData21
  Out1 : Outport
  wires:
  Bus Selector1/2 -> Create nominal q/2(omega)  "<omega>"
  Create nominal q/1(q_nominal) -> Scope6/1, Out1/1
  Bus Selector1/1 -> Create nominal q/1(q)  "<q_est>"
  Create Bus [State Vector,X_a]3/1(X_bus) -> Bus Selector1/1
  In1/1 -> Create Bus [State Vector,X_a]3/1(X)

== system Model_02/Kalman Prediction//Update/Function-Call Subsystem ==
  tr : Inport
  y(0) : Inport  Port=2
  X_a : Inport  Port=3
  function : TriggerPort  TriggerType=function-call  StatesWhenEnabling=reset
  Discrete-Time Integrator2 : DiscreteIntegrator  IntegratorMethod=Integration: Backward Euler  ExternalReset=rising  InitialConditionSource=external  SampleTime=-1  ShowStatePort=on  ICPrevOutput=DiscIntNeverNeededParam  ICPrevScaledInput=DiscIntNeverNeededParam
  Display : Display
  Dynamic Model (Differential equations)2 : Subsystem
  y(t) : Outport
  wires:
  tr/1 -> Discrete-Time Integrator2/2
  y(0)/1 -> Discrete-Time Integrator2/3, Display/1
  Dynamic Model (Differential equations)2/1(X_a_dot) -> Discrete-Time Integrator2/1
  X_a/1 -> Dynamic Model (Differential equations)2/1(X_a(t))
  Discrete-Time Integrator2/1 -> y(t)/1

== system Model_02/Kalman Prediction//Update/Initial Conditions (create bus) ==
  Bus Creator : BusCreator
  Bus Creator1 : BusCreator  Inputs=3
  Bus Creator2 : BusCreator  Inputs=3
  Bus Creator3 : BusCreator  Inputs=3
  Bus Creator4 : BusCreator  NonVirtualBus=on
  Constant : Constant  Value=[X_a_0]
  Demux : Demux  Outputs=13
  Initial conditions (Dynamic Model) : FromFile  FileName=X_a_0_Model_02.mat
  P_post : Constant  Value=eye(12,12)  VectorParams1D=off
  "X_a(0) " : Outport
  "P_post " : Outport  Port=2
  wires:
  Demux/1 -> Bus Creator/1  "q_1"
  Demux/2 -> Bus Creator/2  "q_2"
  Demux/3 -> Bus Creator/3  "q_3"
  Demux/4 -> Bus Creator/4  "q_0"
  Demux/5 -> Bus Creator1/1  "omega_x"
  Demux/6 -> Bus Creator1/2  "omega_y"
  Demux/7 -> Bus Creator1/3  "omega_z"
  Demux/8 -> Bus Creator2/1  "r_x"
  Demux/9 -> Bus Creator2/2  "r_y"
  Demux/10 -> Bus Creator2/3  "r_z"
  Demux/11 -> Bus Creator3/1  "r_x_dot"
  Demux/12 -> Bus Creator3/2  "r_y_dot"
  Demux/13 -> Bus Creator3/3  "r_z_dot"
  Bus Creator/1 -> Bus Creator4/1  "q"
  Bus Creator1/1 -> Bus Creator4/2  "omega"
  Bus Creator2/1 -> Bus Creator4/3  "r"
  Bus Creator3/1 -> Bus Creator4/4  "r_dot"
  Bus Creator4/1 -> "X_a(0) "/1  "X_a(0)"
  P_post/1 -> "P_post "/1
  Constant/1 -> Demux/1

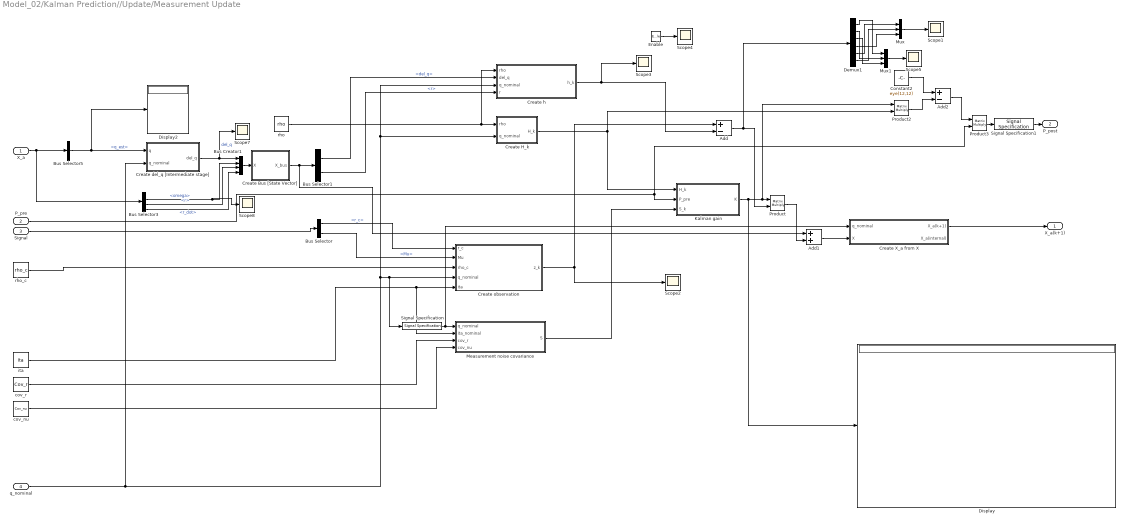
== system Model_02/Kalman Prediction//Update/Measurement Update ==
  X_a : Inport
  P_pre : Inport  Port=2
  Signal : Inport  Port=3
  "q_nominal " : Inport  Port=4
  Enable : EnablePort  ShowOutputPort=on
  Add : Sum  Inputs=+-
  Add1 : Sum
  Add2 : Sum  Inputs=+-
  Bus Creator1 : BusCreator
  Bus Selector : BusSelector  OutputSignals=r_c,Mu
  Bus Selector1 : BusSelector  OutputSignals=del_q,r
  Bus Selector3 : BusSelector  OutputSignals=q_est,omega,r,r_dot
  Bus Selector5 : BusSelector  OutputSignals=q_est
  Constant2 : Constant  Value=eye(12,12)
  Create Bus [State Vector] : Subsystem
  Create H_k : Subsystem
  Create X_a from X : Subsystem
  Create del_q [Intermediate stage] : Subsystem
  Create h : Subsystem
  Create observation : Subsystem
  Demux1 : Demux  Outputs=6
  Display : Display
  Display2 : Display
  Kalman gain : Subsystem
  Measurement noise covariance : MATLAB Function  TreatAsAtomicUnit=on
  Mux : Mux  Inputs=3
  Mux1 : Mux  Inputs=3
  Product : Product  Multiplication=Matrix(*)
  Product2 : Product  Multiplication=Matrix(*)
  Product3 : Product  Multiplication=Matrix(*)
  Scope{1..5,7..8} (7 alike) : Scope
      Scope1 settings: YMin=-0.3  YMax=0.8  SaveName=ScopeData18
      Scope2 settings: SaveName=ScopeData25
      Scope3 settings: SaveName=ScopeData8
      Scope4 settings: SaveName=ScopeData27
      Scope5 settings: SaveName=ScopeData17
      Scope7 settings: TimeRange=40  YMin=-0.045  YMax=0.045  SaveName=ScopeData22
      Scope8 settings: SaveName=ScopeData23
  Signal Specification : SignalSpecification  Dimensions=[4,1]
  Signal Specification1 : SignalSpecification  Dimensions=[12,12]
  cov_nu : Constant  Value=Cov_nu
  cov_r : Constant  Value=Cov_r
  "ita " : Constant  Value=ita
  "rho " : Constant  Value=rho
  rho_c : Constant  Value=rho_c
  X_a(k+1) : Outport
  P_post : Outport  Port=2
  wires:
  Signal/1 -> Bus Selector/1
  Bus Selector/1 -> Create observation/1(r_c)  "<r_c>"
  Bus Selector/2 -> Create observation/2(Mu)  "<Mu>"
  rho_c/1 -> Create observation/3(rho_c)
  "ita "/1 -> Measurement noise covariance/2(ita_nominal), Create observation/5(ita)
  "rho "/1 -> Create h/1(rho), Create H_k/1(rho)
  cov_r/1 -> Measurement noise covariance/3(cov_r)
  cov_nu/1 -> Measurement noise covariance/4(cov_nu)
  Create H_k/1(H_k) -> Kalman gain/1(H_k), Product2/2
  P_pre/1 -> Kalman gain/2(P_pre), Product3/2
  Measurement noise covariance/1(S) -> Kalman gain/3(S_k)
  Bus Selector1/1 -> Create h/2(del_q)  "<del_q>"
  Bus Selector1/2 -> Create h/4(r)  "<r>"
  Create observation/1(z_k) -> Scope2/1, Add/1
  Create h/1(h_k) -> Scope3/1, Add/2
  Kalman gain/1(K) -> Display/1, Product2/1, Product/1
  Add/1 -> Demux1/1, Product/2
  Product/1 -> Add1/2
  Constant2/1 -> Add2/1
  Product2/1 -> Add2/2
  Add2/1 -> Product3/1
  Mux/1 -> Scope1/1
  Demux1/5 -> Mux/1
  Demux1/6 -> Mux/2
  Demux1/4 -> Mux/3
  Signal Specification/1 -> Create X_a from X/1(q_nominal), Measurement noise covariance/1(q_nominal)
  Enable/1 -> Scope4/1
  Product3/1 -> Signal Specification1/1
  Signal Specification1/1 -> P_post/1
  Add1/1 -> Create X_a from X/2(X)
  Create X_a from X/1(X_a(k+1)) -> X_a(k+1)/1
  Demux1/1 -> Mux1/1
  Demux1/2 -> Mux1/2
  Demux1/3 -> Mux1/3
  Mux1/1 -> Scope5/1
  Create del_q [Intermediate stage]/1(del_q) -> Scope7/1, Bus Creator1/1  "del_q"
  Bus Selector3/2 -> Scope8/1, Bus Creator1/2  "<omega>"
  Bus Selector3/3 -> Bus Creator1/3  "<r>"
  Bus Selector3/4 -> Bus Creator1/4  "<r_dot>"
  Bus Creator1/1 -> Create Bus [State Vector]/1(X)
  Bus Selector5/1 -> Display2/1, Create del_q [Intermediate stage]/1(q)  "<q_est>"
  Create Bus [State Vector]/1(X_bus) -> Add1/1, Bus Selector1/1
  X_a/1 -> Bus Selector3/1, Bus Selector5/1
  "q_nominal "/1 -> Create del_q [Intermediate stage]/2(q_nominal), Create h/3(q_nominal), Create H_k/2(q_nominal), Create observation/4(q_nominal), Signal Specification/1

== system Model_02/Kalman Prediction//Update/Process noise covariance [rotational] ==
  Phi : Inport
  Process Noise covariance : MATLAB Function  TreatAsAtomicUnit=on
  p : Constant  Value=[p_x;p_y;p_z]
  sig_tau : Constant  Value=sig_tau
  t_delta : Constant  Value=t_Kalman
  Q_r : Outport
  wires:
  Phi/1 -> Process Noise covariance/1(Phi)
  t_delta/1 -> Process Noise covariance/3(t_delta)
  sig_tau/1 -> Process Noise covariance/4(tau)
  p/1 -> Process Noise covariance/6(p)
  Process Noise covariance/1(Q_r) -> Q_r/1

== system Model_02/Kalman Prediction//Update/Process noise covariance [translational] ==
  Process noise covariance [translational] : MATLAB Function  TreatAsAtomicUnit=on
  n : Constant  Value=n
  sig_f : Constant  Value=sig_f
  t_Kalman : Constant  Value=t_Kalman
  Q_t : Outport
  wires:
  n/1 -> Process noise covariance [translational]/2(n)
  t_Kalman/1 -> Process noise covariance [translational]/1(t_Kalman)
  sig_f/1 -> Process noise covariance [translational]/3(sigma_f)
  Process noise covariance [translational]/1(Q_t_k) -> Q_t/1

== system Model_02/Kalman Prediction//Update/State Propagation ==
  "X_a(t)\t" : Inport
  Create M : Subsystem
  MATLAB Function : MATLAB Function  TreatAsAtomicUnit=on
  n : Constant  Value=n
  p : Constant  Value=[p_x;p_y;p_z]
  "t_Kalman " : Constant  Value=t_Kalman
  Phi : Outport
  wires:
  p/1 -> Create M/2(p), MATLAB Function/4(p)
  n/1 -> MATLAB Function/2(n)
  "t_Kalman "/1 -> MATLAB Function/3(t_Kalman)
  MATLAB Function/1(Phi) -> Phi/1
  "X_a(t)\t"/1 -> Create M/1("X_a "), MATLAB Function/1(X_a)
  Create M/1(M) -> MATLAB Function/5(M)

== system Model_02/Create Measurements [Pose]/Create Measurements [Orientation] /Quaternion norm ==
  q : Inport
  Demux3 : Demux
  Divide{,1..3} (4 alike) : Product  Inputs=*/
  Mux1 : Mux
  Norm(q) : Subsystem
  normalized_q : Outport
  wires:
  Demux3/3 -> Divide2/1
  Norm(q)/1(|q|) -> Divide3/2, Divide2/2, Divide1/2, Divide/2
  Demux3/1 -> Divide/1
  Divide3/1 -> Mux1/4
  Divide2/1 -> Mux1/3
  Mux1/1 -> normalized_q/1
  Demux3/2 -> Divide1/1
  q/1 -> Demux3/1, Norm(q)/1(q)
  Demux3/4 -> Divide3/1
  Divide/1 -> Mux1/1
  Divide1/1 -> Mux1/2

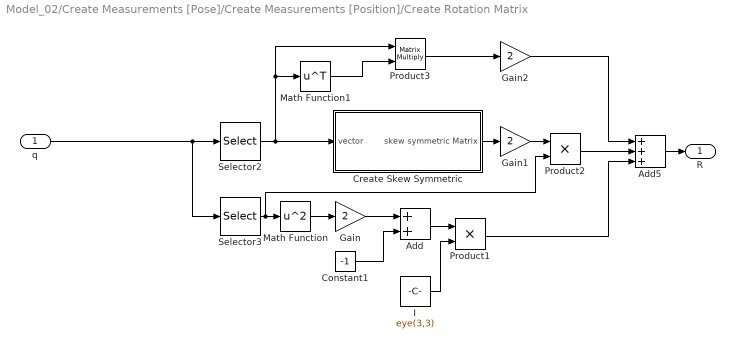
== system Model_02/Create Measurements [Pose]/Create Measurements [Position]/Create Rotation Matrix  ==
  q : Inport
  Add : Sum
  Add5 : Sum  Inputs=+++
  Constant1 : Constant  Value=-1
  Create Skew Symmetric : Subsystem
  Gain : Gain  Gain=2
  Gain1 : Gain  Gain=2
  Gain2 : Gain  Gain=2
  I : Constant  Value=eye(3,3)
  Math Function : Math  Operator=square  SaturateOnIntegerOverflow=on
  Math Function1 : Math  Operator=transpose  SaturateOnIntegerOverflow=on
  Product1 : Product
  Product2 : Product
  Product3 : Product  Multiplication=Matrix(*)
  Selector2 : Selector  NumberOfDimensions=2  InputPortWidth=3  IndexOptions=Index vector (dialog),Index vector (dialog)  Indices=[1 2 3],1  OutputSizes=1,1
  Selector3 : Selector  NumberOfDimensions=2  InputPortWidth=3  IndexOptions=Index vector (dialog),Index vector (dialog)  Indices=[4],1  OutputSizes=1,1
  R : Outport
  wires:
  Gain/1 -> Add/1
  Math Function/1 -> Gain/1
  Constant1/1 -> Add/2
  Selector3/1 -> Product2/2, Math Function/1
  Add/1 -> Product1/1
  I/1 -> Product1/2
  Selector2/1 -> Math Function1/1, Product3/1, Create Skew Symmetric/1(vector)
  Gain2/1 -> Add5/1
  Product2/1 -> Add5/2
  Create Skew Symmetric/1(skew symmetric Matrix) -> Gain1/1
  Gain1/1 -> Product2/1
  Product1/1 -> Add5/3
  Math Function1/1 -> Product3/2
  Product3/1 -> Gain2/1
  Add5/1 -> R/1
  q/1 -> Selector3/1, Selector2/1

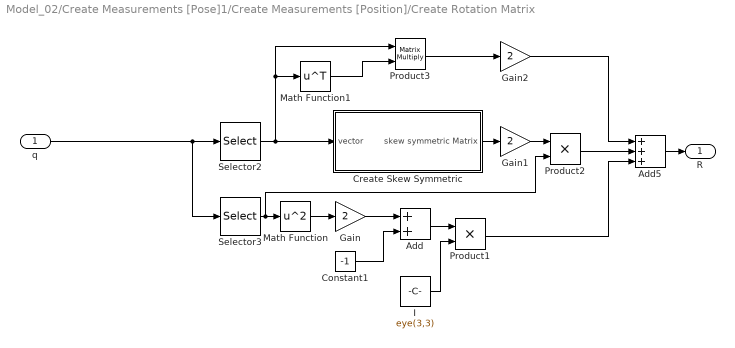
== system Model_02/Create Measurements [Pose]1/Create Measurements [Position]/Create Rotation Matrix  ==
  q : Inport
  Add : Sum
  Add5 : Sum  Inputs=+++
  Constant1 : Constant  Value=-1
  Create Skew Symmetric : Subsystem
  Gain : Gain  Gain=2
  Gain1 : Gain  Gain=2
  Gain2 : Gain  Gain=2
  I : Constant  Value=eye(3,3)
  Math Function : Math  Operator=square  SaturateOnIntegerOverflow=on
  Math Function1 : Math  Operator=transpose  SaturateOnIntegerOverflow=on
  Product1 : Product
  Product2 : Product
  Product3 : Product  Multiplication=Matrix(*)
  Selector2 : Selector  NumberOfDimensions=2  InputPortWidth=3  IndexOptions=Index vector (dialog),Index vector (dialog)  Indices=[1 2 3],1  OutputSizes=1,1
  Selector3 : Selector  NumberOfDimensions=2  InputPortWidth=3  IndexOptions=Index vector (dialog),Index vector (dialog)  Indices=[4],1  OutputSizes=1,1
  R : Outport
  wires:
  q/1 -> Selector2/1, Selector3/1
  Add5/1 -> R/1
  Product3/1 -> Gain2/1
  Math Function1/1 -> Product3/2
  Product1/1 -> Add5/3
  Gain1/1 -> Product2/1
  Create Skew Symmetric/1(skew symmetric Matrix) -> Gain1/1
  Product2/1 -> Add5/2
  Gain2/1 -> Add5/1
  Selector2/1 -> Create Skew Symmetric/1(vector), Product3/1, Math Function1/1
  I/1 -> Product1/2
  Add/1 -> Product1/1
  Selector3/1 -> Math Function/1, Product2/2
  Constant1/1 -> Add/2
  Math Function/1 -> Gain/1
  Gain/1 -> Add/1

== system Model_02/Dynamic Model (Differential equations)/Orbital Dynamics /Create Skew Symmetric ==
  vector : Inport
  0 : Constant  Value=0
  Create 3x3 matrix : Subsystem
  Demux : Demux  Outputs=3
  Demux1 : Demux  Outputs=3
  Gain : Gain  Gain=-1
  skew symmetric Matrix : Outport
  wires:
  0/1 -> Create 3x3 matrix/1(a11), Create 3x3 matrix/5(a22), Create 3x3 matrix/9(a33)
  Demux/3 -> Create 3x3 matrix/2(a12)
  Demux1/2 -> Create 3x3 matrix/3(a13)
  Demux1/3 -> Create 3x3 matrix/4(a21)
  Demux/1 -> Create 3x3 matrix/6(a23)
  vector/1 -> Demux1/1, Gain/1
  Create 3x3 matrix/1(Matrix) -> skew symmetric Matrix/1
  Gain/1 -> Demux/1
  Demux/2 -> Create 3x3 matrix/7(a31)
  Demux1/1 -> Create 3x3 matrix/8(a32)

== system Model_02/Dynamic Model (Differential equations)/Orbital Dynamics /norm  ==
  vector : Inport
  Dot Product : DotProduct  InputSameDT=on  OutDataTypeStr=Inherit: Inherit via internal rule
  Sqrt : Sqrt  SaturateOnIntegerOverflow=on
  "norm " : Outport
  wires:
  Dot Product/1 -> Sqrt/1
  vector/1 -> Dot Product/2, Dot Product/1
  Sqrt/1 -> "norm "/1

== system Model_02/Dynamic Model (Differential equations)/Rotational Dynamics/Create  J ==
  p : Inport
  0 : Constant  Value=0
  1 : Constant
  Create 3x3 matrix : Subsystem
  Fcn : Fcn  Expr=1-u(2)/1+u(1)
  Fcn1 : Fcn  Expr=1+u(3)/1-u(1)
  "J_k " : Outport
  wires:
  Fcn/1 -> Create 3x3 matrix/5(a22)
  p/1 -> Fcn1/1, Fcn/1
  0/1 -> Create 3x3 matrix/2(a12), Create 3x3 matrix/3(a13), Create 3x3 matrix/4(a21), Create 3x3 matrix/6(a23), Create 3x3 matrix/7(a31), Create 3x3 matrix/8(a32)
  Create 3x3 matrix/1(Matrix) -> "J_k "/1
  Fcn1/1 -> Create 3x3 matrix/9(a33)
  1/1 -> Create 3x3 matrix/1(a11)
